simulink model "Mini_Golf_Course"  (R2022a)
settings: Solver=ode23t  StartTime=0.0  StopTime=100  MaxStep=1e-2  RelTol=1e-4  AbsTol=1e-5  EnableMultiTasking=on
PostLoadFcn:
  | % TURN OFF ERROR EXTERNAL FORCE --> WORLD
  | set_param(bdroot,'SimMechanicsRigidlyBoundBlock','none')
  | set_param(bdroot,'IgnoredZcDiagnostic','none')
InitFcn:
  | %% DO NOT CHANGE -- START %%
  | 
  | % GET HOLE NUMBER
  | HoleChoice = get_param([bdroot '/Course'],'ActiveVariant');
  | HoleChoice = strrep(HoleChoice,' ','_');
  | UndSc_ind = findstr(HoleChoice,'_');
  | HoleNum = str2num(HoleChoice(UndSc_ind+1:end));
  | 
  | % SET BALL INITIAL POSITION
  | ball_init_x = eval(['Mini_Golf_Param.' HoleChoice '.Ball_Init_x']);
  | ball_init_y = eval(['Mini_Golf_Param.' HoleChoice '.Ball_Init_y']);
  | 
  | %%  DO NOT CHANGE -- END %%
StartFcn:
  | tic;
StopFcn:
  | Elapsed_Sim_Time = toc;
  | disp(['Elapsed Sim Time = ' num2str(Elapsed_Sim_Time)]);
  | Plot_Hole_Ball_Trajectory
undefined symbols (not defined in the file or in its folder): Mini_Golf_Param, X, Y, Z
libraries: nesl_utility x16, sm_lib x12, Course_Holes_Lib x1, Golf_Components_Lib x1
Description:
  | Mini Golf Course
  | 
  | Copyright 2015-2022 The MathWorks, Inc.
settings Model: Creator=smiller  LastModifiedBy=smiller
settings SolverCC: AutoScaleAbsTol=off  AlgebraicLoopSolver=TrustRegion
settings DataIOCC: SaveFormat=Array  ReturnWorkspaceOutputs=off
settings OptimizationCC: LifeSpan=inf
settings DebuggingCC: IgnoredZcDiagnostic=none  SolverPrmCheckMsg=warning  UnconnectedInputMsg=warning  UnconnectedOutputMsg=warning  UnconnectedLineMsg=warning  AllowSymbolicDim=off  PregeneratedLibrarySubsystemCodeDiagnostic=none  SFUnexpectedBacktrackingDiag=warning  SFNoUnconditionalDefaultTransitionDiag=warning  SFExecutionAtInitializationDiag=none  SFMachineParentedDataDiag=warning  ArithmeticOperatorsInVariantConditions=warning
settings HardwareCC: ProdBitPerPointer=32  ProdBitPerSizeT=32  ProdBitPerPtrDiffT=32  ProdLargestAtomicFloat=None  ProdIntDivRoundTo=Undefined  ProdEndianess=Unspecified  ProdWordSize=32  ProdHWDeviceType=32-bit Generic
settings ModelReferenceCC: PropagateSignalLabelsOutOfModel=off
settings SFSimCC: SimUseLocalCustomCode=off  CustomCodeUndefinedFunction=UseInterfaceOnly
settings RTWCC: RTWUseLocalCustomCode=off  DLArmComputeVersion=19.05
settings CodeAppCC: StateflowObjectComments=on
settings GRTTargetCC: TargetLangStandard=C89/C90 (ANSI)
settings ConfigComp: CovMetricSettings=dw  CovSaveCumulativeToWorkspaceVar=on  CovSaveSingleToWorkspaceVar=on  CovExternalEMLEnable=off  CovSFcnEnable=off
settings SimscapeCC: SimscapeNormalizeSystem=off  SimscapeLogType=all  SimscapeLogName=simlog_Mini_Golf_Course
settings ConfigurationSet: Description=SimMechanics 2G
settings DiagnosticsConfigSet: SimMechanicsRigidlyBoundBlock=none
settings ExplorerConfigSet: InternalSimMechanicsExplorerSettings="<ExplorerConfiguration><canonicalview>default</canonicalview><AnimationSetting><BasePlaybackSpeed>1.0</BasePlaybackSpeed><PlaybackSpeedFactor>2.0</PlaybackSpeedFactor></AnimationSetting><TilePanel><TileInfo><Tiles Columns=\"1\" Count=\"1\" Rows=\"1\"><Column Left=\"2\" Weight=\"1\"/><Column Left=\"677\"/><Row Top=\"2\" Weight=\"1\"/><Row Top=\"558\"/><Tile Height=\"1\" Width=\"1\" X=\"0\" Y=\"0\"/></Tiles></TileInfo><SceneInfo><SceneViewer><BGColor><R>0.92156863212585449</R><G>0.96470588445663452</G><B>0.96470588445663452</B></BGColor><Camera><Position><X>8.3655702861838535</X><Y>-5.3723201545767978</Y><Z>5.3560301548682645</Z></Position><Center><X>2.9932501316070557</X><Y>0</Y><Z>-0.016289999708533287</Z></Center><Up><X>-0.40824829046386307</X><Y>0.40824829046386307</Y><Z>0.81649658092772615</Z></Up><Left>-3.0491064190864563</Left><Right>3.0491064190864563</Right><Bottom>-1.8109499931335451</Bottom><Top>1.8109499931335451</Top></Camera></SceneViewer></SceneInfo></TilePanel></ExplorerConfiguration>"

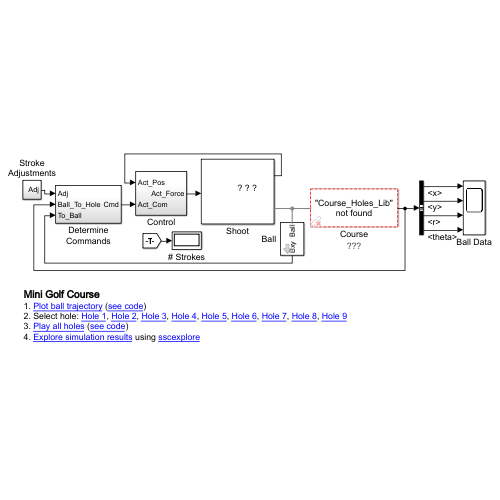
[thumbnail: Simulink's stored preview of the top-level diagram]
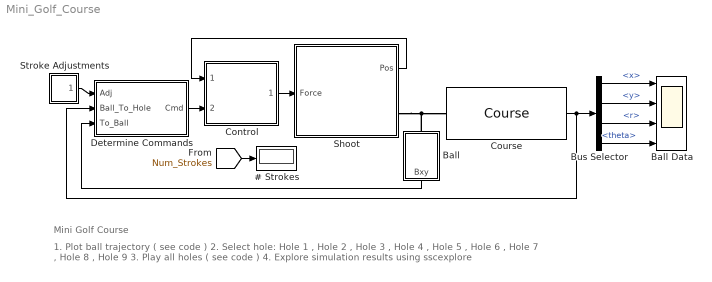
== system Mini_Golf_Course ==
  note: Mini Golf Course
  note: 1. Plot ball trajectory ( see code )
      | 2. Select hole: Hole 1 , Hole 2 , Hole 3 , Hole 4 , Hole 5 , Hole 6 , Hole 7 , Hole 8 , Hole 9
      | 3. Play all holes ( see code )
      | 4. Explore simulation results using sscexplore
  # Strokes : Display
  Ball : Subsystem  mask{init_ball_pos=[ball_init_x ball_init_y], init_ball_vel=[0 0]}
      mask prompts: init_ball_pos "Ball Initial Position [x y] (m)"; init_ball_vel "Ball Initial Velocity [vx vy] (m/s)"
      mask init:
      | init_ball_x = init_ball_pos(1);
      | init_ball_y = init_ball_pos(2);
      | init_ball_vx = init_ball_vel(1);
      | init_ball_vy = init_ball_vel(2);
  Ball Data : Scope  NumInputPorts=4
  Bus Selector : BusSelector  OutputSignals=x,y,r,theta
  Control : Subsystem
  Course : Course_Holes_Lib/Course  SystemSampleTime=-1  LabelModeActiveChoice=Hole_1  VariantActivationTime=update diagram  Latency=0  AutoFrameSizeCalculation=off
      settings: AttributesFormatString=%<BlockChoice>
  Determine Commands : Subsystem
  Shoot : Subsystem
      mask Display:
      | image(imread('Putter_Shoot_IMAGE.jpg'));
      | port_label('input',1,'Force');
      | port_label('output',1,'Pos');
      | port_label('RConn',1,'Putt2Ball');
  Stroke Adjustments : Subsystem
  wires:
  Course/1 -> Bus Selector/1, Determine Commands/2(Ball_To_Hole)
  Bus Selector/1 -> Ball Data/1  "<x>"
  Bus Selector/2 -> Ball Data/2  "<y>"
  Bus Selector/3 -> Ball Data/3  "<r>"
  Bus Selector/4 -> Ball Data/4  "<theta>"
  Ball/1(Bxy) -> Determine Commands/3(To_Ball)
  Determine Commands/1(Cmd) -> Control/2(Act_Com)
  Shoot/1(Pos) -> Control/1(Act_Pos)
  Control/1(Act_Force) -> Shoot/1(Force)
  Stroke Adjustments/1(Adj) -> Determine Commands/1(Adj)
  [Num_Strokes] -> # Strokes/1
  connections:
  Ball/LConn1 -- Course/LConn1 -- Shoot/RConn1

== system Mini_Golf_Course/Ball ==
  Ball Sensing : Subsystem
  Ball Solid : sm_lib/Body Elements/Spherical Solid  GraphicAmbientColor=[0.15 0.15 0.15 1.0]  BasedOnType=Mass  CenterOfMass=[0 0 0]  CenterOfMassUnits=m  GraphicDiffuseColor=[1.0 1.0 1.0]  Density=1000  DensityUnits=kg/(m^3)  DoExposeReferenceFrame=on  GraphicEmissiveColor=[0.0 0.0 0.0 1.0]  ExportEntireGeometry=off  SerializedExposedGeometries=<ExposedGeometries/>  SerializedFrames=<Frames/>  MarkerShape=Sphere  MarkerSize=10  GraphicType=FromGeometry  InertiaType=CalculateFromGeometry  Mass=Mini_Golf_Param.Ball.Mass  MassUnits=g  MomentsOfInertia=[1 1 1]  MomentsOfInertiaUnits=kg*m^2  GraphicOpacity=1.0  ProductsOfInertia=[0 0 0]  ProductsOfInertiaUnits=kg*m^2  GraphicShininess=75  GraphicSpecularColor=[0.5 0.5 0.5 1.0]  SphereRadius=Mini_Golf_Param.Ball.Radius  SphereRadiusUnits=m  GraphicVisPropType=SimpleVisualProperties
  Mechanism Configuration : sm_lib/Utilities/Mechanism Configuration  UniformGravity=Constant  GravityVector=[0 0 -9.81]  GravityUnits=m/s^2  LinearizationDelta=0.001  JointModeTransitionNonlinearIterations=2
  Rectangular Joint : sm_lib/Joints/Rectangular Joint  JointMode=Normal  SenseConstraintForce=off  SenseConstraintForceX=off  SenseConstraintForceY=off  SenseConstraintForceZ=off  SenseConstraintTorque=off  SenseConstraintTorqueX=off  SenseConstraintTorqueY=off  SenseConstraintTorqueZ=off  SenseTotalForce=off  SenseTotalForceX=off  SenseTotalForceY=off  SenseTotalForceZ=off  SenseTotalTorque=off  SenseTotalTorqueX=off  SenseTotalTorqueY=off  SenseTotalTorqueZ=off  CompositeWrenchDir=FollowerOnBase  CompositeWrenchFrame=BaseFrame  PxEquilibriumPosition=0  PxEquilibriumPositionUnits=m  PxSpringStiffness=0  PxSpringStiffnessUnits=N/m  PxDampingCoefficient=Mini_Golf_Param.Ball.Friction  PxDampingCoefficientUnits=N/(m/s)  PxTorqueActuationMode=NoTorque  PxMotionActuationMode=ComputedMotion  PxSensePosition=off  PxSenseVelocity=off  PxSenseAcceleration=off  PxSenseTorqueForce=off  PxSenseLowerLimitTorqueForce=off  PxSenseUpperLimitTorqueForce=off  PxLowerLimitSpecify=off  PxLowerLimitBound=-1  PxLowerLimitBoundUnits=m  PxLowerLimitStiffness=1e6  PxLowerLimitStiffnessUnits=N/m  PxLowerLimitDamping=1e3  PxLowerLimitDampingUnits=N/(m/s)  PxLowerLimitTransitionRegionWidth=1e-4  PxLowerLimitTransitionRegionWidthUnits=m  PxUpperLimitSpecify=off  PxUpperLimitBound=1  PxUpperLimitBoundUnits=m  PxUpperLimitStiffness=1e6  PxUpperLimitStiffnessUnits=N/m  PxUpperLimitDamping=1e3  PxUpperLimitDampingUnits=N/(m/s)  PxUpperLimitTransitionRegionWidth=1e-4  PxUpperLimitTransitionRegionWidthUnits=m  PxPositionTargetSpecify=on  PxPositionTargetPriority=High  PxPositionTargetValue=init_ball_x  PxPositionTargetValueUnits=m  PxVelocityTargetSpecify=on  PxVelocityTargetPriority=High  PxVelocityTargetValue=init_ball_vx  PxVelocityTargetValueUnits=m/s  PyEquilibriumPosition=0  PyEquilibriumPositionUnits=m  PySpringStiffness=0  PySpringStiffnessUnits=N/m  PyDampingCoefficient=Mini_Golf_Param.Ball.Friction  PyDampingCoefficientUnits=N/(m/s)  PyTorqueActuationMode=NoTorque  PyMotionActuationMode=ComputedMotion  PySensePosition=off  PySenseVelocity=off  PySenseAcceleration=off  PySenseTorqueForce=off  PySenseLowerLimitTorqueForce=off  PySenseUpperLimitTorqueForce=off  PyLowerLimitSpecify=off  PyLowerLimitBound=-1  PyLowerLimitBoundUnits=m  PyLowerLimitStiffness=1e6  PyLowerLimitStiffnessUnits=N/m  PyLowerLimitDamping=1e3  PyLowerLimitDampingUnits=N/(m/s)  PyLowerLimitTransitionRegionWidth=1e-4  PyLowerLimitTransitionRegionWidthUnits=m  PyUpperLimitSpecify=off  PyUpperLimitBound=1  PyUpperLimitBoundUnits=m  PyUpperLimitStiffness=1e6  PyUpperLimitStiffnessUnits=N/m  PyUpperLimitDamping=1e3  PyUpperLimitDampingUnits=N/(m/s)  PyUpperLimitTransitionRegionWidth=1e-4  PyUpperLimitTransitionRegionWidthUnits=m  PyPositionTargetSpecify=on  PyPositionTargetPriority=High  PyPositionTargetValue=init_ball_y  PyPositionTargetValueUnits=m  PyVelocityTargetSpecify=on  PyVelocityTargetPriority=High  PyVelocityTargetValue=init_ball_vy  PyVelocityTargetValueUnits=m/s
  Solver Configuration : nesl_utility/Solver Configuration  PhysicalDomain=network_engine_domain  SubClassName=solver  LeftPortType=input  RightPortType=generic  Tones=[]  Harmonics=[]  SimulateNoise=off  Profile=off  UseLocalSampling=off  EnableSwitchedLinearOptims=on  FrequencyDomain=off  UseCCode=off  RelTol=0.001  AbsTol=1e-06  MinStep=1e-09  ToWorkspace=off  RevertToSquareIcSolve=off  NumHomotopyIterations=100  PhasorMode=off  PhasorModeNumHarmonics=1  IndexReductionMethod=DerivativeReplacement  DoDC=off  ResidualTolerance=1e-9  UseLocalSolver=off  LocalSolverChoice=NE_BACKWARD_EULER_ADVANCER  LocalSolverSampleTime=.001  DoFixedCost=off  MaxNonlinIter=3  MaxModeIter=2  ComputeImpulses=off  ImpulseIterations=2  LinearAlgebra=Sparse  LinearAlgebraNumThread=0  EquationFormulation=NE_TIME_EF  DelaysMemoryBudget=1024  AutomaticFiltering=on  FilteringTimeConstant=0.001  PartitionStorageMethod=AS_NEEDED  PartitionMemoryBudget=1024  PartitionMethod=FAST
      settings: SourceProductBaseCode=SS,PW,VE
  World Frame : sm_lib/Frames and Transforms/World Frame
  Ball : PMIOPort  Side=Left
  Bxy : Outport  VectorParamsAs1DForOutWhenUnconnected=off
  wires:
  Ball Sensing/1(Ball_sig) -> Bxy/1
  connections:
  Rectangular Joint/LConn1 -- Mechanism Configuration/RConn1 -- Solver Configuration/RConn1 -- World Frame/RConn1
  Ball Solid/RConn1 -- Ball/RConn1 -- Ball Sensing/LConn1 -- Rectangular Joint/RConn1

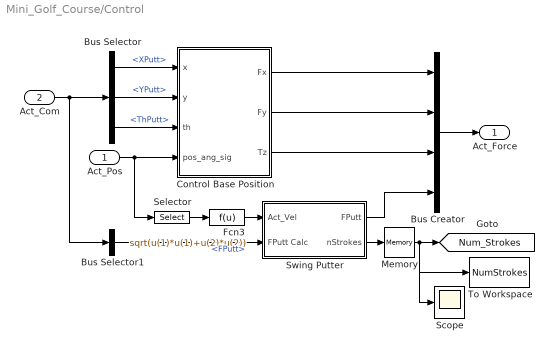
== system Mini_Golf_Course/Control ==
  Act_Pos : Inport
  Act_Com : Inport  Port=2
  Bus Creator : BusCreator  Inputs=4
  Bus Selector : BusSelector  OutputSignals=XPutt,YPutt,ThPutt
  Bus Selector1 : BusSelector  OutputSignals=FPutt
  Control Base Position : Subsystem
  Fcn3 : Fcn  Expr=sqrt(u(1)*u(1)+u(2)*u(2))
  Memory : Memory  InheritSampleTime=on
  Scope : Scope
  Selector : Selector  InputPortWidth=6  IndexOptions=Index vector (dialog)  Indices=[2 4]  OutputSizes=1
  Swing Putter : Subsystem
  To Workspace : ToWorkspace  VariableName=NumStrokes  SampleTime=-1
      settings: MaxDataPoints=1
  Act_Force : Outport  VectorParamsAs1DForOutWhenUnconnected=off
  tag scope: Num_Strokes=global
  wires:
  Act_Pos/1 -> Selector/1, Control Base Position/4(pos_ang_sig)
  Bus Selector/1 -> Control Base Position/1(x)  "<XPutt>"
  Bus Selector/2 -> Control Base Position/2(y)  "<YPutt>"
  Bus Selector/3 -> Control Base Position/3(th)  "<ThPutt>"
  Swing Putter/1(FPutt) -> Bus Creator/4
  Selector/1 -> Fcn3/1
  Fcn3/1 -> Swing Putter/1(Act_Vel)
  Act_Com/1 -> Bus Selector/1, Bus Selector1/1
  Control Base Position/3(Tz) -> Bus Creator/3
  Control Base Position/2(Fy) -> Bus Creator/2
  Control Base Position/1(Fx) -> Bus Creator/1
  Bus Creator/1 -> Act_Force/1
  Swing Putter/2(nStrokes) -> Memory/1
  Bus Selector1/1 -> Swing Putter/2(FPutt Calc)  "<FPutt>"
  Memory/1 -> [Num_Strokes], Scope/1, To Workspace/1

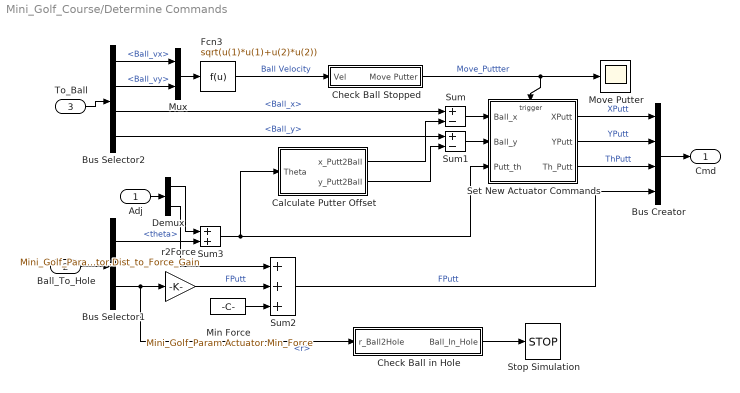
== system Mini_Golf_Course/Determine Commands ==
  Adj : Inport
  Ball_To_Hole : Inport  Port=2
  To_Ball : Inport  Port=3
  Bus Creator : BusCreator  Inputs=4
  Bus Selector1 : BusSelector  OutputSignals=theta,r
  Bus Selector2 : BusSelector  OutputSignals=Ball_vx,Ball_vy,Ball_x,Ball_y
  Calculate Putter Offset : Subsystem
  Check Ball Stopped : Subsystem
  Check Ball in Hole : Subsystem
  Demux : Demux  Outputs=2
  Fcn3 : Fcn  Expr=sqrt(u(1)*u(1)+u(2)*u(2))
  Min Force : Constant  Value=Mini_Golf_Param.Actuator.Min_Force
  Move Putter : Scope
  Mux : Mux  Inputs=2
  Set New Actuator Commands : Subsystem  TreatAsAtomicUnit=on
  Stop Simulation : Stop
  Sum : Sum  Inputs=+-
  Sum1 : Sum  Inputs=+-
  Sum2 : Sum  Inputs=+++
  Sum3 : Sum
  r2Force : Gain  Gain=Mini_Golf_Param.Actuator.Dist_to_Force_Gain
  Cmd : Outport  VectorParamsAs1DForOutWhenUnconnected=off
  wires:
  Ball_To_Hole/1 -> Bus Selector1/1
  To_Ball/1 -> Bus Selector2/1
  Bus Selector2/3 -> Sum/1  "<Ball_x>"
  Bus Selector2/4 -> Sum1/1  "<Ball_y>"
  Bus Selector1/2 -> r2Force/1, Check Ball in Hole/1(r_Ball2Hole)  "<r>"
  Calculate Putter Offset/1(x_Putt2Ball) -> Sum/2
  Calculate Putter Offset/2(y_Putt2Ball) -> Sum1/2
  Sum/1 -> Set New Actuator Commands/1(Ball_x)
  Sum1/1 -> Set New Actuator Commands/2(Ball_y)
  Set New Actuator Commands/1(XPutt) -> Bus Creator/1  "XPutt"
  Set New Actuator Commands/2(YPutt) -> Bus Creator/2  "YPutt"
  Set New Actuator Commands/3(Th_Putt) -> Bus Creator/3  "ThPutt"
  Bus Selector2/1 -> Mux/1  "<Ball_vx>"
  Bus Selector2/2 -> Mux/2  "<Ball_vy>"
  Mux/1 -> Fcn3/1
  Fcn3/1 -> Check Ball Stopped/1(Vel)  "Ball Velocity"
  Check Ball Stopped/1(Move Putter) -> Set New Actuator Commands/Trigger, Move Putter/1  "Move_Puttter"
  Bus Creator/1 -> Cmd/1
  Check Ball in Hole/1(Ball_In_Hole) -> Stop Simulation/1
  r2Force/1 -> Sum2/2  "FPutt"
  Sum2/1 -> Bus Creator/4  "FPutt"
  Adj/1 -> Demux/1
  Min Force/1 -> Sum2/3
  Demux/2 -> Sum2/1
  Sum3/1 -> Set New Actuator Commands/3(Putt_th), Calculate Putter Offset/1(Theta)
  Demux/1 -> Sum3/1
  Bus Selector1/1 -> Sum3/2  "<theta>"

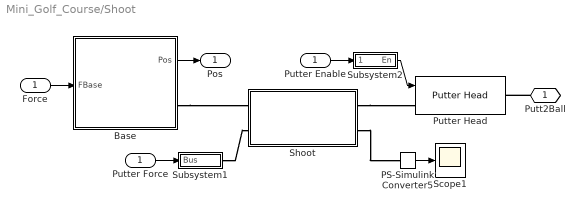
== system Mini_Golf_Course/Shoot ==
  Force : Inport
  Base : Subsystem
      mask Display:
      | image(imread('Base_Shoot_IMAGE.jpg'));
      | port_label('input',1,'FBase');
      | port_label('output',1,'Pos');
      | port_label('RConn',1,'CG');
  PS-Simulink Converter5 : nesl_utility/PS-Simulink Converter  PhysicalDomain=network_engine_domain  SubClassName=ps_output  LeftPortType=input  RightPortType=output  PseudoPeriodic=off  Frequencies=[]  VectorFormat=1-D array  Unit=1  AffineConversion=off
      settings: SourceProductBaseCode=SS,PW,VE
  Putter Enable : InportShadow
  Putter Force : InportShadow
  Putter Head : Golf_Components_Lib/Putter Head  length=Mini_Golf_Param.Putter.Length  height=Mini_Golf_Param.Putter.Height  width=Mini_Golf_Param.Putter.Width  ball_radius=Mini_Golf_Param.Ball.Radius  contact_k=Mini_Golf_Param.Wall.Stiffness  contact_b=Mini_Golf_Param.Wall.Damping  low_pass_filt_const=Mini_Golf_Param.Wall.Low_Pass_Filt_Const
  Scope1 : Scope
  Shoot : Subsystem
      mask Display:
      | image(imread('Shoot_IMAGE.jpg'));
      | port_label('LConn',1,'Actuator');
      | port_label('RConn',1,'Handle');
      | port_label('LConn',2,'Fz');
      | port_label('RConn',2,'p');
  Subsystem1 : Subsystem
  Subsystem2 : Subsystem
  Putt2Ball : PMIOPort  Side=Right
  Pos : Outport  VectorParamsAs1DForOutWhenUnconnected=off
  wires:
  Base/1(Pos) -> Pos/1
  Force/1 -> Base/1(FBase)
  Putter Force/1 -> Subsystem1/1(Bus)
  PS-Simulink Converter5/1 -> Scope1/1
  Putter Enable/1 -> Subsystem2/1(Bus)
  Subsystem2/1(En) -> Putter Head/1
  connections:
  Base/RConn1 -- Shoot/LConn1
  Subsystem1/RConn1 -- Shoot/LConn2
  Shoot/RConn2 -- PS-Simulink Converter5/LConn1
  Putt2Ball/RConn1 -- Putter Head/RConn1
  Shoot/RConn1 -- Putter Head/LConn1

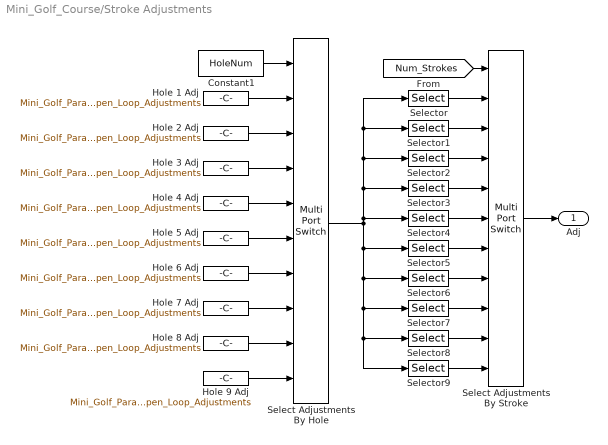
== system Mini_Golf_Course/Stroke Adjustments ==
  Constant1 : Constant  Value=HoleNum
  Hole 1 Adj : Constant  Value=Mini_Golf_Param.Hole_1.Open_Loop_Adjustments
  Hole 2 Adj : Constant  Value=Mini_Golf_Param.Hole_2.Open_Loop_Adjustments
  Hole 3 Adj : Constant  Value=Mini_Golf_Param.Hole_3.Open_Loop_Adjustments
  Hole 4 Adj : Constant  Value=Mini_Golf_Param.Hole_4.Open_Loop_Adjustments
  Hole 5 Adj : Constant  Value=Mini_Golf_Param.Hole_5.Open_Loop_Adjustments
  Hole 6 Adj : Constant  Value=Mini_Golf_Param.Hole_6.Open_Loop_Adjustments
  Hole 7 Adj : Constant  Value=Mini_Golf_Param.Hole_7.Open_Loop_Adjustments
  Hole 8 Adj : Constant  Value=Mini_Golf_Param.Hole_8.Open_Loop_Adjustments
  Hole 9 Adj : Constant  Value=Mini_Golf_Param.Hole_9.Open_Loop_Adjustments
  Select Adjustments By Hole : MultiPortSwitch  Inputs=9  DiagnosticForDefault=None  SaturateOnIntegerOverflow=off  InputSameDT=off
  Select Adjustments By Stroke : MultiPortSwitch  DataPortOrder=Zero-based contiguous  Inputs=10  DiagnosticForDefault=None  zeroidx=on  SaturateOnIntegerOverflow=off  InputSameDT=off
  Selector : Selector  NumberOfDimensions=2  InputPortWidth=3  IndexOptions=Index vector (dialog),Index vector (dialog)  Indices=1,1:2  OutputSizes=1,1
  Selector1 : Selector  NumberOfDimensions=2  InputPortWidth=3  IndexOptions=Index vector (dialog),Index vector (dialog)  Indices=2,1:2  OutputSizes=1,1
  Selector2 : Selector  NumberOfDimensions=2  InputPortWidth=3  IndexOptions=Index vector (dialog),Index vector (dialog)  Indices=3,1:2  OutputSizes=1,1
  Selector3 : Selector  NumberOfDimensions=2  InputPortWidth=3  IndexOptions=Index vector (dialog),Index vector (dialog)  Indices=4,1:2  OutputSizes=1,1
  Selector4 : Selector  NumberOfDimensions=2  InputPortWidth=3  IndexOptions=Index vector (dialog),Index vector (dialog)  Indices=5,1:2  OutputSizes=1,1
  Selector5 : Selector  NumberOfDimensions=2  InputPortWidth=3  IndexOptions=Index vector (dialog),Index vector (dialog)  Indices=6,1:2  OutputSizes=1,1
  Selector6 : Selector  NumberOfDimensions=2  InputPortWidth=3  IndexOptions=Index vector (dialog),Index vector (dialog)  Indices=7,1:2  OutputSizes=1,1
  Selector7 : Selector  NumberOfDimensions=2  InputPortWidth=3  IndexOptions=Index vector (dialog),Index vector (dialog)  Indices=8,1:2  OutputSizes=1,1
  Selector8 : Selector  NumberOfDimensions=2  InputPortWidth=3  IndexOptions=Index vector (dialog),Index vector (dialog)  Indices=9,1:2  OutputSizes=1,1
  Selector9 : Selector  NumberOfDimensions=2  InputPortWidth=3  IndexOptions=Index vector (dialog),Index vector (dialog)  Indices=10,1:2  OutputSizes=1,1
  Adj : Outport  VectorParamsAs1DForOutWhenUnconnected=off
  wires:
  [Num_Strokes] -> Select Adjustments By Stroke/1
  Select Adjustments By Stroke/1 -> Adj/1
  Selector/1 -> Select Adjustments By Stroke/2
  Selector1/1 -> Select Adjustments By Stroke/3
  Selector2/1 -> Select Adjustments By Stroke/4
  Selector3/1 -> Select Adjustments By Stroke/5
  Selector4/1 -> Select Adjustments By Stroke/6
  Selector5/1 -> Select Adjustments By Stroke/7
  Selector6/1 -> Select Adjustments By Stroke/8
  Selector7/1 -> Select Adjustments By Stroke/9
  Selector8/1 -> Select Adjustments By Stroke/10
  Selector9/1 -> Select Adjustments By Stroke/11
  Constant1/1 -> Select Adjustments By Hole/1
  Hole 1 Adj/1 -> Select Adjustments By Hole/2
  Hole 2 Adj/1 -> Select Adjustments By Hole/3
  Select Adjustments By Hole/1 -> Selector/1, Selector1/1, Selector2/1, Selector3/1, Selector4/1, Selector5/1, Selector6/1, Selector7/1, Selector8/1, Selector9/1
  Hole 3 Adj/1 -> Select Adjustments By Hole/4
  Hole 4 Adj/1 -> Select Adjustments By Hole/5
  Hole 5 Adj/1 -> Select Adjustments By Hole/6
  Hole 6 Adj/1 -> Select Adjustments By Hole/7
  Hole 7 Adj/1 -> Select Adjustments By Hole/8
  Hole 8 Adj/1 -> Select Adjustments By Hole/9
  Hole 9 Adj/1 -> Select Adjustments By Hole/10

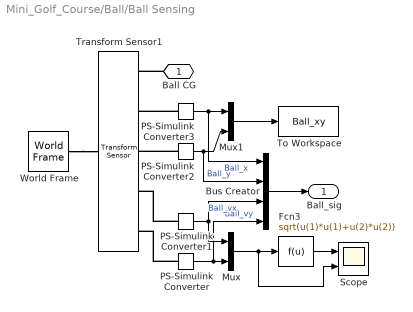
== system Mini_Golf_Course/Ball/Ball Sensing ==
  Bus Creator : BusCreator  Inputs=4
  Fcn3 : Fcn  Expr=sqrt(u(1)*u(1)+u(2)*u(2))
  Mux : Mux  Inputs=2
  Mux1 : Mux  Inputs=2
  PS-Simulink Converter{,1..3} (4 alike) : nesl_utility/PS-Simulink Converter  PhysicalDomain=network_engine_domain  SubClassName=ps_output  LeftPortType=input  RightPortType=output  PseudoPeriodic=off  Frequencies=[]  VectorFormat=1-D array  Unit=1  AffineConversion=off
      settings: SourceProductBaseCode=SS,PW,VE
  Scope : Scope  NumInputPorts=2
  To Workspace : ToWorkspace  VariableName=Ball_xy  SaveFormat=Structure  SampleTime=-1
  Transform Sensor1 : sm_lib/Frames and Transforms/Transform Sensor  MeasurementFrame=World  SenseAngle=off  SenseAxis=off  SenseAngle1=off  SenseAngle2=off  SenseAngle3=off  SenseQ=off  SenseR=off  SenseOmegaX=off  SenseOmegaY=off  SenseOmegaZ=off  SenseOmega1=off  SenseOmega2=off  SenseOmega3=off  SenseQDot=off  SenseRDot=off  SenseAlphaX=off  SenseAlphaY=off  SenseAlphaZ=off  SenseAlpha1=off  SenseAlpha2=off  SenseAlpha3=off  SenseQDDot=off  SenseRDDot=off  SenseX=on  SenseY=on  SenseZ=off  SenseRad=off  SenseAzim=off  SenseDist=off  SenseInc=off  SenseXDot=on  SenseYDot=on  SenseZDot=off  SenseRadDot=off  SenseAzimDot=off  SenseDistDot=off  SenseIncDot=off  SenseXDDot=off  SenseYDDot=off  SenseZDDot=off  SenseRadDDot=off  SenseAzimDDot=off  SenseDistDDot=off  SenseIncDDot=off
  World Frame : sm_lib/Frames and Transforms/World Frame
  Ball CG : PMIOPort  Side=Left
  Ball_sig : Outport  VectorParamsAs1DForOutWhenUnconnected=off
  wires:
  PS-Simulink Converter/1 -> Mux/2, Bus Creator/4  "Ball_vy"
  Mux/1 -> Fcn3/1, Scope/2
  PS-Simulink Converter1/1 -> Mux/1, Bus Creator/3  "Ball_vx"
  Fcn3/1 -> Scope/1
  PS-Simulink Converter3/1 -> Mux1/1, Bus Creator/1  "Ball_x"
  PS-Simulink Converter2/1 -> Mux1/2, Bus Creator/2  "Ball_y"
  Mux1/1 -> To Workspace/1
  Bus Creator/1 -> Ball_sig/1
  connections:
  PS-Simulink Converter/LConn1 -- Transform Sensor1/RConn5
  PS-Simulink Converter1/LConn1 -- Transform Sensor1/RConn4
  PS-Simulink Converter2/LConn1 -- Transform Sensor1/RConn3
  PS-Simulink Converter3/LConn1 -- Transform Sensor1/RConn2
  World Frame/RConn1 -- Transform Sensor1/LConn1
  Ball CG/RConn1 -- Transform Sensor1/RConn1

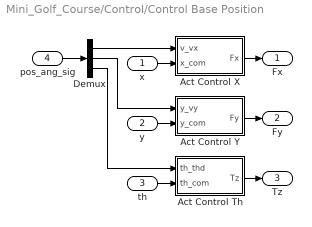
== system Mini_Golf_Course/Control/Control Base Position ==
  x : Inport
  y : Inport  Port=2
  th : Inport  Port=3
  pos_ang_sig : Inport  Port=4
  Act Control Th : Subsystem
  Act Control X : Subsystem
  Act Control Y : Subsystem
  Demux : Demux  Outputs=3
  Fx : Outport  VectorParamsAs1DForOutWhenUnconnected=off
  Fy : Outport  Port=2  VectorParamsAs1DForOutWhenUnconnected=off
  Tz : Outport  Port=3  VectorParamsAs1DForOutWhenUnconnected=off
  wires:
  pos_ang_sig/1 -> Demux/1
  Demux/1 -> Act Control X/1(v_vx)
  Act Control X/1(Fx) -> Fx/1
  y/1 -> Act Control Y/2(y_com)
  Act Control Y/1(Fy) -> Fy/1
  Demux/2 -> Act Control Y/1(y_vy)
  Act Control Th/1(Tz) -> Tz/1
  Demux/3 -> Act Control Th/1(th_thd)
  x/1 -> Act Control X/2(x_com)
  th/1 -> Act Control Th/2(th_com)

== system Mini_Golf_Course/Control/Swing Putter ==
  Act_Vel : Inport
  FPutt Calc : Inport  Port=2
  Actuator Stopped : Scope  NumInputPorts=2
  Check Actuator Stopped : Subsystem
  Create Force Pulse : Subsystem
  Triggered Subsystem : Subsystem  TreatAsAtomicUnit=on
  FPutt : Outport  VectorParamsAs1DForOutWhenUnconnected=off
  nStrokes : Outport  Port=2  VectorParamsAs1DForOutWhenUnconnected=off
  wires:
  Create Force Pulse/1(Force Pulse) -> FPutt/1
  Act_Vel/1 -> Check Actuator Stopped/1(Act_Vel), Actuator Stopped/1
  FPutt Calc/1 -> Triggered Subsystem/1(FPutt Calc)
  Check Actuator Stopped/1(Swing Putter) -> Triggered Subsystem/Trigger, Create Force Pulse/1(Reset Force), Actuator Stopped/2
  Triggered Subsystem/2(Num_Strokes) -> nStrokes/1
  Triggered Subsystem/1(FPutt Cmd) -> Create Force Pulse/2(Putt Force)

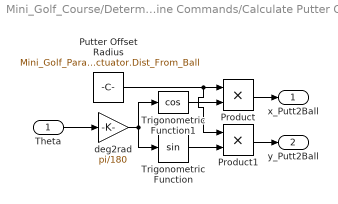
== system Mini_Golf_Course/Determine Commands/Calculate Putter Offset ==
  Theta : Inport
  Product : Product  RndMeth=Zero
  Product1 : Product  RndMeth=Zero
  Putter Offset Radius : Constant  Value=Mini_Golf_Param.Actuator.Dist_From_Ball
  Trigonometric Function : Trigonometry
  Trigonometric Function1 : Trigonometry  Operator=cos
  deg2rad : Gain  Gain=pi/180
  x_Putt2Ball : Outport  VectorParamsAs1DForOutWhenUnconnected=off
  y_Putt2Ball : Outport  Port=2  VectorParamsAs1DForOutWhenUnconnected=off
  wires:
  deg2rad/1 -> Trigonometric Function/1, Trigonometric Function1/1
  Trigonometric Function1/1 -> Product/2
  Trigonometric Function/1 -> Product1/2
  Putter Offset Radius/1 -> Product/1, Product1/1
  Theta/1 -> deg2rad/1
  Product/1 -> x_Putt2Ball/1
  Product1/1 -> y_Putt2Ball/1

== system Mini_Golf_Course/Determine Commands/Check Ball Stopped ==
  Vel : Inport
  Ball Velocity Threshold : Constant  Value=Mini_Golf_Param.Logic.Ball_Stopped_Vel_Thresh
  "Min Time at Rest " : Delay  DelayLength=Mini_Golf_Param.Logic.Ball_Stopped_Samples  SampleTime=Mini_Golf_Param.Logic.Ball_Stopped_Sample_Time
  Product1 : Product  OutDataTypeStr=double  RndMeth=Zero
  Relational Operator1 : RelationalOperator  Operator=<=  OutDataTypeStr=boolean  InputSameDT=off
  Move Putter : Outport  VectorParamsAs1DForOutWhenUnconnected=off
  wires:
  "Min Time at Rest "/1 -> Product1/1
  Product1/1 -> Move Putter/1
  Relational Operator1/1 -> Product1/2, "Min Time at Rest "/1
  Ball Velocity Threshold/1 -> Relational Operator1/2
  Vel/1 -> Relational Operator1/1

== system Mini_Golf_Course/Determine Commands/Check Ball in Hole ==
  r_Ball2Hole : Inport
  Distance Threshold : Constant  Value=Mini_Golf_Param.Ball.Radius
  Product1 : Product  OutDataTypeStr=double  RndMeth=Zero
  Relational Operator : RelationalOperator  Operator=<=  OutDataTypeStr=boolean  InputSameDT=off
  Time Within Range : Delay  DelayLength=Mini_Golf_Param.Logic.Ball_In_Hole_Samples  SampleTime=Mini_Golf_Param.Logic.Ball_In_Hole_Sample_Time
  Ball_In_Hole : Outport  VectorParamsAs1DForOutWhenUnconnected=off
  wires:
  Product1/1 -> Ball_In_Hole/1
  Time Within Range/1 -> Product1/1
  Distance Threshold/1 -> Relational Operator/2
  Relational Operator/1 -> Time Within Range/1, Product1/2
  r_Ball2Hole/1 -> Relational Operator/1

== system Mini_Golf_Course/Determine Commands/Set New Actuator Commands ==
  note: Triggered Subsystem used to keep commanded position
      | of putter constant while the ball is moving.
  Ball_x : Inport
  Ball_y : Inport  Port=2
  Putt_th : Inport  Port=3
  Trigger : TriggerPort  VariantControl=Variant
  XPutt : Outport  VectorParamsAs1DForOutWhenUnconnected=off
  YPutt : Outport  Port=2  VectorParamsAs1DForOutWhenUnconnected=off
  Th_Putt : Outport  Port=3  VectorParamsAs1DForOutWhenUnconnected=off
  wires:
  Ball_x/1 -> XPutt/1
  Ball_y/1 -> YPutt/1
  Putt_th/1 -> Th_Putt/1

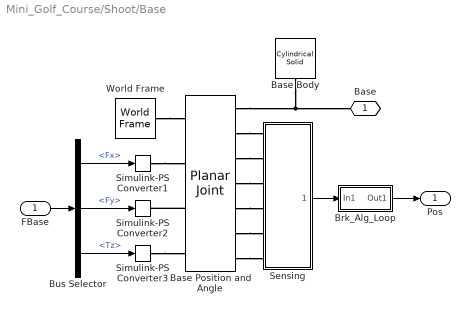
== system Mini_Golf_Course/Shoot/Base ==
  FBase : Inport
  Base Body : sm_lib/Body Elements/Cylindrical Solid  GraphicAmbientColor=[0.15 0.15 0.15 1.0]  BasedOnType=Mass  CenterOfMass=[0 0 0]  CenterOfMassUnits=m  GraphicDiffuseColor=[0.6 0.6 1.0]  CylinderLength=Mini_Golf_Param.Putter.Height*0.5  CylinderLengthUnits=m  CylinderRadius=Mini_Golf_Param.Putter.Length*0.5  CylinderRadiusUnits=m  Density=1000  DensityUnits=kg/(m^3)  DoExposeReferenceFrame=on  GraphicEmissiveColor=[0.0 0.0 0.0 1.0]  ExportEntireGeometry=off  SerializedFrames=<Frames/>  MarkerShape=Sphere  MarkerSize=10  GraphicType=FromGeometry  InertiaType=CalculateFromGeometry  Mass=Mini_Golf_Param.Actuator.Mass  MassUnits=kg  MomentsOfInertia=[1 1 1]  MomentsOfInertiaUnits=kg*m^2  GraphicOpacity=1.0  ProductsOfInertia=[0 0 0]  ProductsOfInertiaUnits=kg*m^2  GraphicShininess=75  GraphicSpecularColor=[0.5 0.5 0.5 1.0]  GraphicVisPropType=SimpleVisualProperties
  Base Position and Angle : sm_lib/Joints/Planar Joint  JointMode=Normal  SenseConstraintForce=off  SenseConstraintForceX=off  SenseConstraintForceY=off  SenseConstraintForceZ=off  SenseConstraintTorque=off  SenseConstraintTorqueX=off  SenseConstraintTorqueY=off  SenseConstraintTorqueZ=off  SenseTotalForce=off  SenseTotalForceX=off  SenseTotalForceY=off  SenseTotalForceZ=off  SenseTotalTorque=off  SenseTotalTorqueX=off  SenseTotalTorqueY=off  SenseTotalTorqueZ=off  CompositeWrenchDir=FollowerOnBase  CompositeWrenchFrame=BaseFrame  PxEquilibriumPosition=0  PxEquilibriumPositionUnits=m  PxSpringStiffness=0  PxSpringStiffnessUnits=N/m  PxDampingCoefficient=Mini_Golf_Param.Actuator.Damping_x  PxDampingCoefficientUnits=N/(m/s)  PxTorqueActuationMode=InputTorque  PxMotionActuationMode=ComputedMotion  PxSensePosition=on  PxSenseVelocity=on  PxSenseAcceleration=off  PxSenseTorqueForce=off  PxSenseLowerLimitTorqueForce=off  PxSenseUpperLimitTorqueForce=off  PxLowerLimitSpecify=off  PxLowerLimitBound=-1  PxLowerLimitBoundUnits=m  PxLowerLimitStiffness=1e6  PxLowerLimitStiffnessUnits=N/m  PxLowerLimitDamping=1e3  PxLowerLimitDampingUnits=N/(m/s)  PxLowerLimitTransitionRegionWidth=1e-4  PxLowerLimitTransitionRegionWidthUnits=m  PxUpperLimitSpecify=off  PxUpperLimitBound=1  PxUpperLimitBoundUnits=m  PxUpperLimitStiffness=1e6  PxUpperLimitStiffnessUnits=N/m  PxUpperLimitDamping=1e3  PxUpperLimitDampingUnits=N/(m/s)  PxUpperLimitTransitionRegionWidth=1e-4  PxUpperLimitTransitionRegionWidthUnits=m  PxPositionTargetSpecify=off  PxPositionTargetPriority=High  PxPositionTargetValue=0  PxPositionTargetValueUnits=m  PxVelocityTargetSpecify=off  PxVelocityTargetPriority=High  PxVelocityTargetValue=0  PxVelocityTargetValueUnits=m/s  PyEquilibriumPosition=0  PyEquilibriumPositionUnits=m  PySpringStiffness=0  PySpringStiffnessUnits=N/m  PyDampingCoefficient=Mini_Golf_Param.Actuator.Damping_y  PyDampingCoefficientUnits=N/(m/s)  PyTorqueActuationMode=InputTorque  PyMotionActuationMode=ComputedMotion  PySensePosition=on  PySenseVelocity=on  PySenseAcceleration=off  PySenseTorqueForce=off  PySenseLowerLimitTorqueForce=off  PySenseUpperLimitTorqueForce=off  PyLowerLimitSpecify=off  PyLowerLimitBound=-1  PyLowerLimitBoundUnits=m  PyLowerLimitStiffness=1e6  PyLowerLimitStiffnessUnits=N/m  PyLowerLimitDamping=1e3  PyLowerLimitDampingUnits=N/(m/s)  PyLowerLimitTransitionRegionWidth=1e-4  PyLowerLimitTransitionRegionWidthUnits=m  PyUpperLimitSpecify=off  PyUpperLimitBound=1  PyUpperLimitBoundUnits=m  PyUpperLimitStiffness=1e6  PyUpperLimitStiffnessUnits=N/m  PyUpperLimitDamping=1e3  PyUpperLimitDampingUnits=N/(m/s)  PyUpperLimitTransitionRegionWidth=1e-4  PyUpperLimitTransitionRegionWidthUnits=m  PyPositionTargetSpecify=off  PyPositionTargetPriority=High  PyPositionTargetValue=0  PyPositionTargetValueUnits=m  PyVelocityTargetSpecify=off  PyVelocityTargetPriority=High  PyVelocityTargetValue=0  PyVelocityTargetValueUnits=m/s  RzEquilibriumPosition=0  RzEquilibriumPositionUnits=rad  RzSpringStiffness=0  RzSpringStiffnessUnits=N*m/rad  RzDampingCoefficient=Mini_Golf_Param.Actuator.Damping_az  RzDampingCoefficientUnits=N*m/(rad/s)  RzTorqueActuationMode=InputTorque  RzMotionActuationMode=ComputedMotion  RzSensePosition=on  RzSenseVelocity=on  RzSenseAcceleration=off  RzSenseTorqueForce=off  RzSenseLowerLimitTorqueForce=off  RzSenseUpperLimitTorqueForce=off  RzLowerLimitSpecify=off  RzLowerLimitBound=-90  RzLowerLimitBoundUnits=deg  RzLowerLimitStiffness=1e4  RzLowerLimitStiffnessUnits=N*m/deg  RzLowerLimitDamping=10  RzLowerLimitDampingUnits=N*m/(deg/s)  RzLowerLimitTransitionRegionWidth=0.1  RzLowerLimitTransitionRegionWidthUnits=deg  RzUpperLimitSpecify=off  RzUpperLimitBound=90  RzUpperLimitBoundUnits=deg  RzUpperLimitStiffness=1e4  RzUpperLimitStiffnessUnits=N*m/deg  RzUpperLimitDamping=10  RzUpperLimitDampingUnits=N*m/(deg/s)  RzUpperLimitTransitionRegionWidth=0.1  RzUpperLimitTransitionRegionWidthUnits=deg  RzPositionTargetSpecify=off  RzPositionTargetPriority=High  RzPositionTargetValue=0  RzPositionTargetValueUnits=rad  RzVelocityTargetSpecify=off  RzVelocityTargetPriority=High  RzVelocityTargetValue=0  RzVelocityTargetValueUnits=rad/s
  Brk_Alg_Loop : Subsystem  mask(First-order lag supporting vector signals){b=Mini_Golf_Param.Actuator.Low_Pass_Filter_Constant, x_initial=0}
      mask prompts: b "Filter time constant"; x_initial "Initial output"
      mask help: Models a lag of the form 1/(b*s+1) where s is the Laplace operator.
  Bus Selector : BusSelector  OutputSignals=Fx,Fy,Tz
  Sensing : Subsystem
  Simulink-PS Converter1 : nesl_utility/Simulink-PS Converter  PhysicalDomain=network_engine_domain  SubClassName=ps_input  LeftPortType=input  RightPortType=output  PseudoPeriodic=off  Frequencies=[]  NoiseDistribution=none  NoiseParameters=[]  Unit=1  AffineConversion=off  FilteringAndDerivatives=zero  SimscapeFilterOrder=1  InputFilterTimeConstant=0.005  UdotUserProvided=[]
      settings: SourceProductBaseCode=SS,PW,VE
  Simulink-PS Converter2 : nesl_utility/Simulink-PS Converter  PhysicalDomain=network_engine_domain  SubClassName=ps_input  LeftPortType=input  RightPortType=output  PseudoPeriodic=off  Frequencies=[]  NoiseDistribution=none  NoiseParameters=[]  Unit=1  AffineConversion=off  FilteringAndDerivatives=zero  SimscapeFilterOrder=1  InputFilterTimeConstant=0.005  UdotUserProvided=[]
      settings: SourceProductBaseCode=SS,PW,VE
  Simulink-PS Converter3 : nesl_utility/Simulink-PS Converter  PhysicalDomain=network_engine_domain  SubClassName=ps_input  LeftPortType=input  RightPortType=output  PseudoPeriodic=off  Frequencies=[]  NoiseDistribution=none  NoiseParameters=[]  Unit=1  AffineConversion=off  FilteringAndDerivatives=zero  SimscapeFilterOrder=1  InputFilterTimeConstant=0.005  UdotUserProvided=[]
      settings: SourceProductBaseCode=SS,PW,VE
  World Frame : sm_lib/Frames and Transforms/World Frame
  Base : PMIOPort  Side=Right
  Pos : Outport  VectorParamsAs1DForOutWhenUnconnected=off
  wires:
  FBase/1 -> Bus Selector/1
  Brk_Alg_Loop/1(Out1) -> Pos/1
  Sensing/1(pos_ang_sig) -> Brk_Alg_Loop/1(In1)
  Bus Selector/1 -> Simulink-PS Converter1/1  "<Fx>"
  Bus Selector/2 -> Simulink-PS Converter2/1  "<Fy>"
  Bus Selector/3 -> Simulink-PS Converter3/1  "<Tz>"
  connections:
  Base Position and Angle/RConn7 -- Sensing/LConn6
  Base Position and Angle/RConn6 -- Sensing/LConn5
  Base Position and Angle/RConn5 -- Sensing/LConn4
  Base Position and Angle/RConn4 -- Sensing/LConn3
  Base Position and Angle/RConn3 -- Sensing/LConn2
  Base Position and Angle/RConn2 -- Sensing/LConn1
  Simulink-PS Converter3/RConn1 -- Base Position and Angle/LConn4
  Base Position and Angle/LConn3 -- Simulink-PS Converter2/RConn1
  Simulink-PS Converter1/RConn1 -- Base Position and Angle/LConn2
  World Frame/RConn1 -- Base Position and Angle/LConn1
  Base Body/RConn1 -- Base Position and Angle/RConn1 -- Base/RConn1

== system Mini_Golf_Course/Shoot/Shoot ==
  Handle Actuator Transform : sm_lib/Frames and Transforms/Rigid Transform  TranslationMethod=None  TranslationStandardOffset=0  TranslationLengthUnit=m  TranslationStandardAxis=+Z  TranslationCartesianOffset=[0 0 0]  TranslationROffset=0  TranslationROffsetUnits=m  TranslationZOffset=0  TranslationZOffsetUnits=m  TranslationThetaOffset=0  TranslationThetaOffsetUnits=deg  RotationMethod=StandardAxis  RotationAngleUnits=deg  RotationStandardAxis=+Y  RotationAngle=90  RotationArbitraryAxis=[0 0 1]  FollAlignAxisA=+X  BaseAlignAxisA=+Y  FollAlignAxisB=+Y  BaseAlignAxisB=+Z  RotationSequenceAxes=FollowerAxes  RotationSequence=XYX  RotationSequenceAngles=[0 0 0]  RotationSequenceAnglesUnits=deg  RotationMatrix=[1 0 0; 0 1 0; 0 0 1]
  Putter Actuation : sm_lib/Joints/Prismatic Joint  JointMode=Normal  SenseConstraintForce=off  SenseConstraintForceX=off  SenseConstraintForceY=off  SenseConstraintForceZ=off  SenseConstraintTorque=off  SenseConstraintTorqueX=off  SenseConstraintTorqueY=off  SenseConstraintTorqueZ=off  SenseTotalForce=off  SenseTotalForceX=off  SenseTotalForceY=off  SenseTotalForceZ=off  SenseTotalTorque=off  SenseTotalTorqueX=off  SenseTotalTorqueY=off  SenseTotalTorqueZ=off  CompositeWrenchDir=FollowerOnBase  CompositeWrenchFrame=BaseFrame  EquilibriumPosition=0  EquilibriumPositionUnits=m  SpringStiffness=Mini_Golf_Param.Actuator.Putter_Spring_k  SpringStiffnessUnits=N/m  DampingCoefficient=Mini_Golf_Param.Actuator.Putter_Damper_b  DampingCoefficientUnits=N/(m/s)  TorqueActuationMode=InputTorque  MotionActuationMode=ComputedMotion  SensePosition=on  SenseVelocity=off  SenseAcceleration=off  SenseTorqueForce=off  SenseLowerLimitTorqueForce=off  SenseUpperLimitTorqueForce=off  LowerLimitSpecify=off  LowerLimitBound=-1  LowerLimitBoundUnits=m  LowerLimitStiffness=1e6  LowerLimitStiffnessUnits=N/m  LowerLimitDamping=1e3  LowerLimitDampingUnits=N/(m/s)  LowerLimitTransitionRegionWidth=1e-4  LowerLimitTransitionRegionWidthUnits=m  UpperLimitSpecify=off  UpperLimitBound=1  UpperLimitBoundUnits=m  UpperLimitStiffness=1e6  UpperLimitStiffnessUnits=N/m  UpperLimitDamping=1e3  UpperLimitDampingUnits=N/(m/s)  UpperLimitTransitionRegionWidth=1e-4  UpperLimitTransitionRegionWidthUnits=m  PositionTargetSpecify=off  PositionTargetPriority=High  PositionTargetValue=0  PositionTargetValueUnits=m  VelocityTargetSpecify=off  VelocityTargetPriority=High  VelocityTargetValue=0  VelocityTargetValueUnits=m/s
  Putter Handle Transform : sm_lib/Frames and Transforms/Rigid Transform  TranslationMethod=None  TranslationStandardOffset=0  TranslationLengthUnit=m  TranslationStandardAxis=+Z  TranslationCartesianOffset=[0 0 0]  TranslationROffset=0  TranslationROffsetUnits=m  TranslationZOffset=0  TranslationZOffsetUnits=m  TranslationThetaOffset=0  TranslationThetaOffsetUnits=deg  RotationMethod=StandardAxis  RotationAngleUnits=deg  RotationStandardAxis=+Y  RotationAngle=-90  RotationArbitraryAxis=[0 0 1]  FollAlignAxisA=+X  BaseAlignAxisA=+Y  FollAlignAxisB=+Y  BaseAlignAxisB=+Z  RotationSequenceAxes=FollowerAxes  RotationSequence=XYX  RotationSequenceAngles=[0 0 0]  RotationSequenceAnglesUnits=deg  RotationMatrix=[1 0 0; 0 1 0; 0 0 1]
  Base : PMIOPort  Side=Left
  Handle : PMIOPort  Port=2  Side=Right
  Fz : PMIOPort  Port=3  Side=Left
  p : PMIOPort  Port=4  Side=Right
  connections:
  p/RConn1 -- Putter Actuation/RConn2
  Fz/RConn1 -- Putter Actuation/LConn2
  Handle/RConn1 -- Putter Handle Transform/RConn1
  Base/RConn1 -- Handle Actuator Transform/LConn1
  Putter Handle Transform/LConn1 -- Putter Actuation/RConn1
  Handle Actuator Transform/RConn1 -- Putter Actuation/LConn1

== system Mini_Golf_Course/Shoot/Subsystem1 ==
  Bus : Inport
  Bus Selector1 : BusSelector  OutputSignals=FPutt
  Scope1 : Scope
  Simulink-PS Converter : nesl_utility/Simulink-PS Converter  PhysicalDomain=network_engine_domain  SubClassName=ps_input  LeftPortType=input  RightPortType=output  PseudoPeriodic=off  Frequencies=[]  NoiseDistribution=none  NoiseParameters=[]  Unit=1  AffineConversion=off  FilteringAndDerivatives=zero  SimscapeFilterOrder=1  InputFilterTimeConstant=0.005  UdotUserProvided=[]
      settings: SourceProductBaseCode=SS,PW,VE
  F : PMIOPort  Side=Right
  wires:
  Bus Selector1/1 -> Simulink-PS Converter/1, Scope1/1  "<FPutt>"
  Bus/1 -> Bus Selector1/1
  connections:
  F/RConn1 -- Simulink-PS Converter/RConn1

== system Mini_Golf_Course/Shoot/Subsystem2 ==
  Bus : Inport
  Abs : Abs  SaturateOnIntegerOverflow=off
  Bus Selector1 : BusSelector  OutputSignals=FPutt
  Sign : Signum
  En : Outport  VectorParamsAs1DForOutWhenUnconnected=off
  wires:
  Bus/1 -> Bus Selector1/1
  Abs/1 -> Sign/1
  Bus Selector1/1 -> Abs/1  "<FPutt>"
  Sign/1 -> En/1

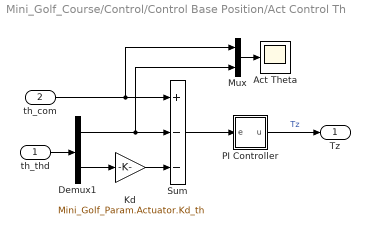
== system Mini_Golf_Course/Control/Control Base Position/Act Control Th ==
  th_thd : Inport
  th_com : Inport  Port=2
  Act Theta : Scope
  Demux1 : Demux  Outputs=2
  Kd : Gain  Gain=Mini_Golf_Param.Actuator.Kd_th
  Mux : Mux  Inputs=2
  PI Controller : Subsystem
      mask Display: disp('PI')
  Sum : Sum  Inputs=+--
  Tz : Outport  VectorParamsAs1DForOutWhenUnconnected=off
  wires:
  Demux1/1 -> Sum/2, Mux/2
  Demux1/2 -> Kd/1
  th_thd/1 -> Demux1/1
  Kd/1 -> Sum/3
  th_com/1 -> Sum/1, Mux/1
  Sum/1 -> PI Controller/1(e)
  PI Controller/1(u) -> Tz/1  "Tz"
  Mux/1 -> Act Theta/1

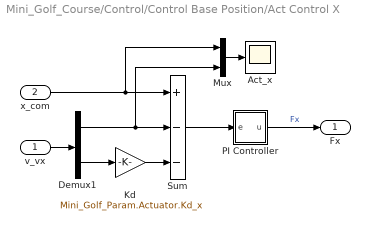
== system Mini_Golf_Course/Control/Control Base Position/Act Control X ==
  v_vx : Inport
  x_com : Inport  Port=2
  Act_x : Scope
  Demux1 : Demux  Outputs=2
  Kd : Gain  Gain=Mini_Golf_Param.Actuator.Kd_x
  Mux : Mux  Inputs=2
  PI Controller : Subsystem
      mask Display: disp('PI')
  Sum : Sum  Inputs=+--
  Fx : Outport  VectorParamsAs1DForOutWhenUnconnected=off
  wires:
  Demux1/1 -> Sum/2, Mux/2
  Demux1/2 -> Kd/1
  v_vx/1 -> Demux1/1
  Kd/1 -> Sum/3
  x_com/1 -> Sum/1, Mux/1
  Sum/1 -> PI Controller/1(e)
  PI Controller/1(u) -> Fx/1  "Fx"
  Mux/1 -> Act_x/1

== system Mini_Golf_Course/Control/Control Base Position/Act Control Y ==
  y_vy : Inport
  y_com : Inport  Port=2
  Act_y : Scope
  Demux1 : Demux  Outputs=2
  Kd : Gain  Gain=Mini_Golf_Param.Actuator.Kd_y
  Mux : Mux  Inputs=2
  PI Controller : Subsystem
      mask Display: disp('PI')
  Sum : Sum  Inputs=+--
  Fy : Outport  VectorParamsAs1DForOutWhenUnconnected=off
  wires:
  Mux/1 -> Act_y/1
  PI Controller/1(u) -> Fy/1  "Fy"
  Sum/1 -> PI Controller/1(e)
  y_com/1 -> Mux/1, Sum/1
  Kd/1 -> Sum/3
  y_vy/1 -> Demux1/1
  Demux1/2 -> Kd/1
  Demux1/1 -> Mux/2, Sum/2

== system Mini_Golf_Course/Control/Swing Putter/Check Actuator Stopped ==
  Act_Vel : Inport
  Actuator Velocity Threshold : Constant  Value=Mini_Golf_Param.Logic.Act_Stopped_Vel_Thresh
  Min Time at Rest : Delay  DelayLength=Mini_Golf_Param.Logic.Act_Stopped_Samples  SampleTime=Mini_Golf_Param.Logic.Act_Stopped_Sample_Time
  Product1 : Product  OutDataTypeStr=double  RndMeth=Zero
  Relational Operator1 : RelationalOperator  Operator=<=  OutDataTypeStr=boolean  InputSameDT=off
  Swing Putter : Outport  VectorParamsAs1DForOutWhenUnconnected=off
  wires:
  Min Time at Rest/1 -> Product1/1
  Product1/1 -> Swing Putter/1
  Relational Operator1/1 -> Min Time at Rest/1, Product1/2
  Actuator Velocity Threshold/1 -> Relational Operator1/2
  Act_Vel/1 -> Relational Operator1/1

== system Mini_Golf_Course/Control/Swing Putter/Create Force Pulse ==
  Reset Force : Inport
  Putt Force : Inport  Port=2
  Delay : Delay  DelayLength=Mini_Golf_Param.Actuator.Force_Samples  ExternalReset=Rising  SampleTime=Mini_Golf_Param.Actuator.Force_Sample_Time
      settings: InputPortMap=u0,r5
  Sum2 : Sum  Inputs=|-+  InputSameDT=on  SaturateOnIntegerOverflow=on  OutDataTypeStr=Inherit: Same as first input
  Force Pulse : Outport  VectorParamsAs1DForOutWhenUnconnected=off
  wires:
  Delay/1 -> Sum2/1
  Putt Force/1 -> Sum2/2, Delay/1
  Reset Force/1 -> Delay/2
  Sum2/1 -> Force Pulse/1  "FPutt"

== system Mini_Golf_Course/Control/Swing Putter/Triggered Subsystem ==
  note: Triggered Subsystem used to set commanded force
      | for the putter once the actuator has stopped moving.
  FPutt Calc : Inport
  Trigger : TriggerPort  VariantControl=Variant
  Memory : Memory  InheritSampleTime=on
  Stroke Increment : Constant
  Sum : Sum  Inputs=|++
  FPutt Cmd : Outport  VectorParamsAs1DForOutWhenUnconnected=off
  Num_Strokes : Outport  Port=2  VectorParamsAs1DForOutWhenUnconnected=off
  wires:
  FPutt Calc/1 -> FPutt Cmd/1
  Stroke Increment/1 -> Sum/2
  Sum/1 -> Num_Strokes/1, Memory/1
  Memory/1 -> Sum/1

== system Mini_Golf_Course/Shoot/Base/Brk_Alg_Loop ==
  In1 : Inport
  Gain : Gain  Gain=1/b
  Integrator : Integrator  InitialCondition=x_initial
  Sum : Sum  Inputs=|+-  InputSameDT=on  SaturateOnIntegerOverflow=on  OutDataTypeStr=Inherit: Same as first input
  Out1 : Outport  VectorParamsAs1DForOutWhenUnconnected=off
  wires:
  Gain/1 -> Out1/1, Sum/2
  Integrator/1 -> Gain/1
  Sum/1 -> Integrator/1
  In1/1 -> Sum/1

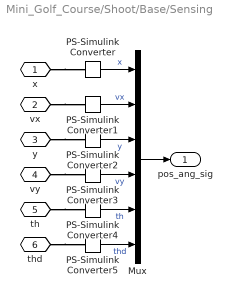
== system Mini_Golf_Course/Shoot/Base/Sensing ==
  Mux : Mux  Inputs=6
  PS-Simulink Converter{,1..3} (4 alike) : nesl_utility/PS-Simulink Converter  PhysicalDomain=network_engine_domain  SubClassName=ps_output  LeftPortType=input  RightPortType=output  PseudoPeriodic=off  Frequencies=[]  VectorFormat=1-D array  Unit=1  AffineConversion=off
      settings: SourceProductBaseCode=SS,PW,VE
  PS-Simulink Converter4 : nesl_utility/PS-Simulink Converter  PhysicalDomain=network_engine_domain  SubClassName=ps_output  LeftPortType=input  RightPortType=output  PseudoPeriodic=off  Frequencies=[]  VectorFormat=1-D array  Unit=deg  AffineConversion=off
      settings: SourceProductBaseCode=SS,PW,VE
  PS-Simulink Converter5 : nesl_utility/PS-Simulink Converter  PhysicalDomain=network_engine_domain  SubClassName=ps_output  LeftPortType=input  RightPortType=output  PseudoPeriodic=off  Frequencies=[]  VectorFormat=1-D array  Unit=deg/s  AffineConversion=off
      settings: SourceProductBaseCode=SS,PW,VE
  x : PMIOPort  Side=Left
  vx : PMIOPort  Port=2  Side=Left
  y : PMIOPort  Port=3  Side=Left
  vy : PMIOPort  Port=4  Side=Left
  th : PMIOPort  Port=5  Side=Left
  thd : PMIOPort  Port=6  Side=Left
  pos_ang_sig : Outport  VectorParamsAs1DForOutWhenUnconnected=off
  wires:
  PS-Simulink Converter5/1 -> Mux/6  "thd"
  PS-Simulink Converter4/1 -> Mux/5  "th"
  Mux/1 -> pos_ang_sig/1
  PS-Simulink Converter3/1 -> Mux/4  "vy"
  PS-Simulink Converter2/1 -> Mux/3  "y"
  PS-Simulink Converter1/1 -> Mux/2  "vx"
  PS-Simulink Converter/1 -> Mux/1  "x"
  connections:
  thd/RConn1 -- PS-Simulink Converter5/LConn1
  th/RConn1 -- PS-Simulink Converter4/LConn1
  vy/RConn1 -- PS-Simulink Converter3/LConn1
  y/RConn1 -- PS-Simulink Converter2/LConn1
  vx/RConn1 -- PS-Simulink Converter1/LConn1
  x/RConn1 -- PS-Simulink Converter/LConn1

== system Mini_Golf_Course/Control/Control Base Position/Act Control Th/PI Controller ==
  e : Inport
  Integral Gain : Gain  Gain=Mini_Golf_Param.Actuator.Ki_th  SaturateOnIntegerOverflow=on  OutDataTypeStr=Inherit: Same as input  ParamDataTypeStr=Inherit: Same as input
  Integrator : Integrator
  Proportional Gain : Gain  Gain=Mini_Golf_Param.Actuator.Kp_th  SaturateOnIntegerOverflow=on  OutDataTypeStr=Inherit: Same as input  ParamDataTypeStr=Inherit: Same as input
  Sum : Sum  Inputs=++|  InputSameDT=on  SaturateOnIntegerOverflow=on  OutDataTypeStr=Inherit: Same as first input
  u : Outport  InitialOutput=0  VectorParamsAs1DForOutWhenUnconnected=off
  wires:
  Sum/1 -> u/1
  e/1 -> Integral Gain/1, Proportional Gain/1
  Integrator/1 -> Sum/2
  Proportional Gain/1 -> Sum/1
  Integral Gain/1 -> Integrator/1

== system Mini_Golf_Course/Control/Control Base Position/Act Control X/PI Controller ==
  e : Inport
  Integral Gain : Gain  Gain=Mini_Golf_Param.Actuator.Ki_x  SaturateOnIntegerOverflow=on  OutDataTypeStr=Inherit: Same as input  ParamDataTypeStr=Inherit: Same as input
  Integrator : Integrator
  Proportional Gain : Gain  Gain=Mini_Golf_Param.Actuator.Kp_x  SaturateOnIntegerOverflow=on  OutDataTypeStr=Inherit: Same as input  ParamDataTypeStr=Inherit: Same as input
  Sum : Sum  Inputs=++|  InputSameDT=on  SaturateOnIntegerOverflow=on  OutDataTypeStr=Inherit: Same as first input
  u : Outport  InitialOutput=0  VectorParamsAs1DForOutWhenUnconnected=off
  wires:
  Sum/1 -> u/1
  e/1 -> Integral Gain/1, Proportional Gain/1
  Integrator/1 -> Sum/2
  Proportional Gain/1 -> Sum/1
  Integral Gain/1 -> Integrator/1

== system Mini_Golf_Course/Control/Control Base Position/Act Control Y/PI Controller ==
  e : Inport
  Integral Gain : Gain  Gain=Mini_Golf_Param.Actuator.Ki_y  SaturateOnIntegerOverflow=on  OutDataTypeStr=Inherit: Same as input  ParamDataTypeStr=Inherit: Same as input
  Integrator : Integrator
  Proportional Gain : Gain  Gain=Mini_Golf_Param.Actuator.Kp_y  SaturateOnIntegerOverflow=on  OutDataTypeStr=Inherit: Same as input  ParamDataTypeStr=Inherit: Same as input
  Sum : Sum  Inputs=++|  InputSameDT=on  SaturateOnIntegerOverflow=on  OutDataTypeStr=Inherit: Same as first input
  u : Outport  InitialOutput=0  VectorParamsAs1DForOutWhenUnconnected=off
  wires:
  Integral Gain/1 -> Integrator/1
  Proportional Gain/1 -> Sum/1
  Integrator/1 -> Sum/2
  e/1 -> Proportional Gain/1, Integral Gain/1
  Sum/1 -> u/1
